simulink model "BasicAudio_Target"  (R2022b)
settings: Solver=FixedStepDiscrete  StartTime=0.0  StopTime=1  RelTol=1e-3  EnableMultiTasking=on
InitFcn:
  | % Initialize model
  | run([ ModelRootName() 'Init.m' ]);
  | 
  | % load library data
  | GainLibrary_data;
  | % Load saved values from partition process
  | TOP_Mask.LoadMapFromFile(bdroot)
model workspace (MAT data in the model file):
  PreampVolumeTable_Idx : Simulink.Signal (value not decoded)
  Range : Simulink.Signal (value not decoded)
  Table_Idx : Simulink.Signal (value not decoded)
undefined symbols (not defined in the file or in its folder): ModelCfg, RgainBusUtil
libraries: TOP x27, HandyTextFile x14, FeaturePath x7, SetDsm x6, RTC x5, AudioStats x3, CapturedConstLib x3, EdgePorts x2, MuteRamperBtc x1, RgainyBtc x1, simulink_need_slupdate x1, dspsrcs4 x1
(part 4 of 5)

== system BasicAudio_Target/BasicAudio/Treble/Tone/InnerLink/TuneVarOffset ==
  TOP : TOP/TOP  TriggerInit=[440 20 585 80]  TopName=Offset  DataTypeOut=single  BankNumber=BankNumber  PreOverlay=PreOverlay  PostOverlay=PostOverlay  CompatibilityString=[]  Role=Automatic
      settings: SourceProductName=Bose Talaria
  TrivialTranslation : Subsystem  mask(Talaria Trivial Translation){TriggerInit=[300 28 350 72]}
      mask prompts: TriggerInit "Hidden: MoveFcn redraw"
      mask help: A trivial translator connects to a TuneVar on the input side and to a TOP (Target Overlay Parameter) for output. The translator then simply copies the value from TuneVar to TOP with no changes.
      mask init:
      | TrivialTranslationMask.Init(gcbh);
      settings: MoveFcn=TrivialTranslationMask.CB_TriggerInit(gcbh);
      mask Callback TriggerInit: TrivialTranslationMask.CB_TriggerInit(gcbh);
      mask Display:
      | % retrieve icon definition
      | [path,w,h] = TrivialTranslationMask.Icon();
      | 
      | % retrieve the block's pixel size
      | pos = get(gcbh,'position');
      | bw = pos(3) - pos(1);
      | bh = pos(4) - pos(2);
      | 
      | % draw centered icon
      | xAdj = bw/2 - w/2;
      | yAdj = bh/2 - h/2;
      | for i=1:length(path)
      |    patch(path(i).x+xAdj, path(i).y+yAdj, path(i).rgb);
      | end
      | disp('COPY   ');
  Out1 : Outport  VectorParamsAs1DForOutWhenUnconnected=off
  wires:
  TOP/1 -> Out1/1  "variable"

== system BasicAudio_Target/BasicAudio/Treble/Tone/InnerLink/TuneVarRampTime ==
  TOP : TOP/TOP  TriggerInit=[440 20 585 80]  TopName=ramptime  DataTypeOut=single  BankNumber=BankNumber  PreOverlay=PreOverlay  PostOverlay=PostOverlay  CompatibilityString=[]  Role=Automatic
      settings: SourceProductName=Bose Talaria
  TrivialTranslation : Subsystem  mask(Talaria Trivial Translation){TriggerInit=[300 28 350 72]}
      mask prompts: TriggerInit "Hidden: MoveFcn redraw"
      mask help: A trivial translator connects to a TuneVar on the input side and to a TOP (Target Overlay Parameter) for output. The translator then simply copies the value from TuneVar to TOP with no changes.
      mask init:
      | TrivialTranslationMask.Init(gcbh);
      settings: MoveFcn=TrivialTranslationMask.CB_TriggerInit(gcbh);
      mask Callback TriggerInit: TrivialTranslationMask.CB_TriggerInit(gcbh);
      mask Display:
      | % retrieve icon definition
      | [path,w,h] = TrivialTranslationMask.Icon();
      | 
      | % retrieve the block's pixel size
      | pos = get(gcbh,'position');
      | bw = pos(3) - pos(1);
      | bh = pos(4) - pos(2);
      | 
      | % draw centered icon
      | xAdj = bw/2 - w/2;
      | yAdj = bh/2 - h/2;
      | for i=1:length(path)
      |    patch(path(i).x+xAdj, path(i).y+yAdj, path(i).rgb);
      | end
      | disp('COPY   ');
  Out1 : Outport  VectorParamsAs1DForOutWhenUnconnected=off
  wires:
  TOP/1 -> Out1/1  "variable"

== system BasicAudio_Target/BasicAudio/Treble/Tone/InnerLink/TuneVarScale ==
  TOP : TOP/TOP  TriggerInit=[440 20 585 80]  TopName=Scale  DataTypeOut=single  BankNumber=BankNumber  PreOverlay=PreOverlay  PostOverlay=PostOverlay  CompatibilityString=[]  Role=Automatic
      settings: SourceProductName=Bose Talaria
  TrivialTranslation : Subsystem  mask(Talaria Trivial Translation){TriggerInit=[300 28 350 72]}
      mask prompts: TriggerInit "Hidden: MoveFcn redraw"
      mask help: A trivial translator connects to a TuneVar on the input side and to a TOP (Target Overlay Parameter) for output. The translator then simply copies the value from TuneVar to TOP with no changes.
      mask init:
      | TrivialTranslationMask.Init(gcbh);
      settings: MoveFcn=TrivialTranslationMask.CB_TriggerInit(gcbh);
      mask Callback TriggerInit: TrivialTranslationMask.CB_TriggerInit(gcbh);
      mask Display:
      | % retrieve icon definition
      | [path,w,h] = TrivialTranslationMask.Icon();
      | 
      | % retrieve the block's pixel size
      | pos = get(gcbh,'position');
      | bw = pos(3) - pos(1);
      | bh = pos(4) - pos(2);
      | 
      | % draw centered icon
      | xAdj = bw/2 - w/2;
      | yAdj = bh/2 - h/2;
      | for i=1:length(path)
      |    patch(path(i).x+xAdj, path(i).y+yAdj, path(i).rgb);
      | end
      | disp('COPY   ');
  Out1 : Outport  VectorParamsAs1DForOutWhenUnconnected=off
  wires:
  TOP/1 -> Out1/1  "variable"

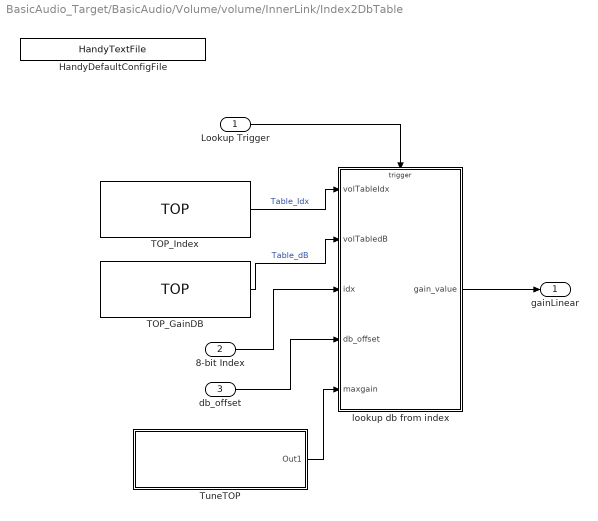
== system BasicAudio_Target/BasicAudio/Volume/volume/InnerLink/Index2DbTable ==
  Lookup Trigger : Inport
  8-bit Index : Inport  Port=2
  db_offset : Inport  Port=3
  HandyDefaultConfigFile : HandyTextFile/HandyTextFile  TemplateSource=Config  FileSuffix=Init  OpenDialogOnLoad=off  UseThisBlockName=off  AddGrandParentNamePrefix=off  TheDefaultText=|  ShowInLibBrowser=on
      | % $(FILENAME) Setup model parameters for each "Init" callback (e.g. update diagram)
      | sample_rate_in_hertz = 44100;
      | frame_size = 32;
      | sysin_channel_count = 2;
      settings: SourceProductName=Bose Talaria
  TOP_GainDB : TOP/TOP  TriggerInit=[635 177 785 233]  TopName=Table_dB  DataTypeOut=Inherit: Same as input  BankNumber=Config.BankNumber  PreOverlay=false  PostOverlay=false  CompatibilityString=[]  Role=Automatic
      settings: SourceProductName=Bose Talaria
  TOP_Index : TOP/TOP  TriggerInit=[635 97 785 153]  TopName=Table_Idx  DataTypeOut=Inherit: Same as input  BankNumber=Config.BankNumber  PreOverlay=false  PostOverlay=false  CompatibilityString=[]  Role=Automatic
      settings: SourceProductName=Bose Talaria
  TuneTOP : Subsystem  Description=Variable limits the maximum *dB offset* which will be applied to the gain as part of table lookup. It does *not* directly impact the maximum gain applied, only the maximum dB offset.  mask(Talaria Trivial Tune TOP){TriggerInit=[670 347 840 403], TopName=maxgain, DataTypeOut=single, BankNumber=0, PreOverlay=false, PostOverlay=false, UseSameName=on}
      mask prompts: TriggerInit "Hidden: MoveFcn redraw"; TopName "Name:"; DataTypeOut "Data type:"; BankNumber "Target memory bank number:"; PreOverlay "Requires pre-overlay action:"; PostOverlay "Requires post-overlay action:"; UseSameName "Use same name for tune variable and TOP"
      mask help: The TuneTOP block encapsultes a Target Overlay Parameter, a Tune Variable, and a Trivial Translation between them.
      mask init:
      | [ok,activeTopPath,activeTunePath] = TuneTOP_Mask.Init(gcbh);
      settings: MoveFcn=TuneTOP_Mask.CB_TriggerInit(gcbh);
      mask Callback TriggerInit: TuneTOP_Mask.CB_TriggerInit(gcbh);
      mask TypeOptions TopName: TOP/TopName
      mask TypeOptions DataTypeOut: TOP/DataTypeOut
      mask TypeOptions BankNumber: TOP/BankNumber
      mask TypeOptions PreOverlay: TOP/PreOverlay
      mask TypeOptions PostOverlay: TOP/PostOverlay
      mask Callback UseSameName: TuneTOP_Mask.CB_UseSameName(gcbh);
      mask DialogControl toolPanel Prompt: Tuning Tool Hints
      mask DialogControl DescriptionGroup Prompt: Description
      mask DialogControl DescriptionText Prompt: Variable limits the maximum *dB offset* which will be applied to the gain as part of table lookup. It does *not* directly impact the maximum gain applied, only the maximum dB offset.
      mask DialogControl EditDescription Prompt: Edit Description
      mask DialogControl EditDescription Callback: TuneTOP_Mask.CB_EditDescription(gcbh);
      mask DialogControl TunabilityText Prompt: Easy: Changes nearly every tuning.
      mask DialogControl AdvancedPanel Prompt: Advanced
      mask DialogControl ConvertToFullTranslation Prompt: Irreversible conversion to full translation
      mask DialogControl ConvertToFullTranslation Callback: TuneTOP_Mask.CB_ConvertToFullTranslation(gcbh);
      mask DialogControl ErrorContainer Prompt: Error Messages
      mask Display:
      | % retrieve icon definition
      | [path,w,h] = TuneTOP_Mask.Icon();
      | 
      | % retrieve the block's pixel size
      | pos = get(gcbh,'position');
      | bw = pos(3) - pos(1);
      | bh = pos(4) - pos(2);
      | 
      | % draw centered icon
      | xAdj = bw/2 - w/2 + 5;
      | yAdj = bh/2 - h/2 + 4;
      | for i=1:length(path)
      | 	patch(path(i).x+xAdj, path(i).y+yAdj, path(i).rgb);
      | end
      | 
      | % show the top name or an X
      | if (exist('ok','var') && ok)
      | 	text(bw*0.5, bh*0.2, activeTopPath, 'horizontalAlignment', 'center');
      | 	patch(0,0,[1 1 1]);
      | 	patch(bw,bh,[1 1 1]);
      | else
      | 	tx=bw*0.03;
      | 	ty=bh*0.03;
      | 	patch([0 tx bw bw-tx], [ty 0 bh-ty bh], [1 0 0]);
      | 	patch([0 bw-tx bw tx], [bh-ty 0 ty bh], [1 0 0]);
      | end
  lookup db from index : MATLAB Function  TreatAsAtomicUnit=on
  gainLinear : Outport  VectorParamsAs1DForOutWhenUnconnected=off
  wires:
  TuneTOP/1(Out1) -> lookup db from index/5(maxgain)
  db_offset/1 -> lookup db from index/4(db_offset)
  TOP_GainDB/1 -> lookup db from index/2(volTabledB)  "Table_dB"
  TOP_Index/1 -> lookup db from index/1(volTableIdx)  "Table_Idx"
  lookup db from index/1(gain_value) -> gainLinear/1
  Lookup Trigger/1 -> lookup db from index/Trigger
  8-bit Index/1 -> lookup db from index/3(idx)

== system BasicAudio_Target/BasicAudio/Volume/volume/InnerLink/Triggered Subsystem ==
  In1 : Inport
  Trigger : TriggerPort  TriggerType=function-call  VariantControl=Variant
  Out1 : Outport
  wires:
  In1/1 -> Out1/1

== system BasicAudio_Target/BasicAudio/Volume/volume/InnerLink/TuneVarRampTimeMs ==
  TOP : TOP/TOP  TriggerInit=[440 20 585 80]  TopName=RampTime  DataTypeOut=single  BankNumber=BankNumber  PreOverlay=PreOverlay  PostOverlay=PostOverlay  CompatibilityString=[]  Role=Automatic
      settings: SourceProductName=Bose Talaria
  TrivialTranslation : Subsystem  mask(Talaria Trivial Translation){TriggerInit=[300 28 350 72]}
      mask prompts: TriggerInit "Hidden: MoveFcn redraw"
      mask help: A trivial translator connects to a TuneVar on the input side and to a TOP (Target Overlay Parameter) for output. The translator then simply copies the value from TuneVar to TOP with no changes.
      mask init:
      | TrivialTranslationMask.Init(gcbh);
      settings: MoveFcn=TrivialTranslationMask.CB_TriggerInit(gcbh);
      mask Callback TriggerInit: TrivialTranslationMask.CB_TriggerInit(gcbh);
      mask Display:
      | % retrieve icon definition
      | [path,w,h] = TrivialTranslationMask.Icon();
      | 
      | % retrieve the block's pixel size
      | pos = get(gcbh,'position');
      | bw = pos(3) - pos(1);
      | bh = pos(4) - pos(2);
      | 
      | % draw centered icon
      | xAdj = bw/2 - w/2;
      | yAdj = bh/2 - h/2;
      | for i=1:length(path)
      |    patch(path(i).x+xAdj, path(i).y+yAdj, path(i).rgb);
      | end
      | disp('COPY   ');
  Out1 : Outport  VectorParamsAs1DForOutWhenUnconnected=off
  wires:
  TOP/1 -> Out1/1  "variable"

== system BasicAudio_Target/BasicAudio/Balance/balance/InnerLink/TuneVarBoostDisable/TrivialTranslation ==

== system BasicAudio_Target/BasicAudio/Balance/balance/InnerLink/TuneVarOffset/TrivialTranslation ==

== system BasicAudio_Target/BasicAudio/Balance/balance/InnerLink/TuneVarRampTime/TrivialTranslation ==

== system BasicAudio_Target/BasicAudio/Balance/balance/InnerLink/TuneVarSilentBass/TrivialTranslation ==

== system BasicAudio_Target/BasicAudio/Balance/balance/InnerLink/TuneVarSilentExtreme/TrivialTranslation ==

== system BasicAudio_Target/BasicAudio/Bass/Tone/InnerLink/TuneVarOffset/TrivialTranslation ==

== system BasicAudio_Target/BasicAudio/Bass/Tone/InnerLink/TuneVarRampTime/TrivialTranslation ==

== system BasicAudio_Target/BasicAudio/Bass/Tone/InnerLink/TuneVarScale/TrivialTranslation ==

== system BasicAudio_Target/BasicAudio/Mute/mute/InnerLink/MuteControl/Triggered Subsystem ==
  In1 : Inport
  Trigger : TriggerPort  TriggerType=function-call  VariantControl=Variant
  Out1 : Outport
  wires:
  In1/1 -> Out1/1

== system BasicAudio_Target/BasicAudio/Mute/mute/InnerLink/MuteControl/TuneVarRampTime ==
  TOP : TOP/TOP  TriggerInit=[440 20 585 80]  TopName=RampTime  DataTypeOut=single  BankNumber=BankNumber  PreOverlay=PreOverlay  PostOverlay=PostOverlay  CompatibilityString=[]  Role=Automatic
      settings: SourceProductName=Bose Talaria
  TrivialTranslation : Subsystem  mask(Talaria Trivial Translation){TriggerInit=[300 28 350 72]}
      mask prompts: TriggerInit "Hidden: MoveFcn redraw"
      mask help: A trivial translator connects to a TuneVar on the input side and to a TOP (Target Overlay Parameter) for output. The translator then simply copies the value from TuneVar to TOP with no changes.
      mask init:
      | TrivialTranslationMask.Init(gcbh);
      settings: MoveFcn=TrivialTranslationMask.CB_TriggerInit(gcbh);
      mask Callback TriggerInit: TrivialTranslationMask.CB_TriggerInit(gcbh);
      mask Display:
      | % retrieve icon definition
      | [path,w,h] = TrivialTranslationMask.Icon();
      | 
      | % retrieve the block's pixel size
      | pos = get(gcbh,'position');
      | bw = pos(3) - pos(1);
      | bh = pos(4) - pos(2);
      | 
      | % draw centered icon
      | xAdj = bw/2 - w/2;
      | yAdj = bh/2 - h/2;
      | for i=1:length(path)
      |    patch(path(i).x+xAdj, path(i).y+yAdj, path(i).rgb);
      | end
      | disp('COPY   ');
  Out1 : Outport  VectorParamsAs1DForOutWhenUnconnected=off
  wires:
  TOP/1 -> Out1/1  "variable"

== system BasicAudio_Target/BasicAudio/Treble/Tone/InnerLink/TuneVarOffset/TrivialTranslation ==

== system BasicAudio_Target/BasicAudio/Treble/Tone/InnerLink/TuneVarRampTime/TrivialTranslation ==

== system BasicAudio_Target/BasicAudio/Treble/Tone/InnerLink/TuneVarScale/TrivialTranslation ==

== system BasicAudio_Target/BasicAudio/Volume/volume/InnerLink/Index2DbTable/TuneTOP ==
  TOP : TOP/TOP  TriggerInit=[440 20 585 80]  TopName=maxgain  DataTypeOut=single  BankNumber=BankNumber  PreOverlay=PreOverlay  PostOverlay=PostOverlay  CompatibilityString=[]  Role=Automatic
      settings: SourceProductName=Bose Talaria
  TrivialTranslation : Subsystem  mask(Talaria Trivial Translation){TriggerInit=[300 28 350 72]}
      mask prompts: TriggerInit "Hidden: MoveFcn redraw"
      mask help: A trivial translator connects to a TuneVar on the input side and to a TOP (Target Overlay Parameter) for output. The translator then simply copies the value from TuneVar to TOP with no changes.
      mask init:
      | TrivialTranslationMask.Init(gcbh);
      settings: MoveFcn=TrivialTranslationMask.CB_TriggerInit(gcbh);
      mask Callback TriggerInit: TrivialTranslationMask.CB_TriggerInit(gcbh);
      mask Display:
      | % retrieve icon definition
      | [path,w,h] = TrivialTranslationMask.Icon();
      | 
      | % retrieve the block's pixel size
      | pos = get(gcbh,'position');
      | bw = pos(3) - pos(1);
      | bh = pos(4) - pos(2);
      | 
      | % draw centered icon
      | xAdj = bw/2 - w/2;
      | yAdj = bh/2 - h/2;
      | for i=1:length(path)
      |    patch(path(i).x+xAdj, path(i).y+yAdj, path(i).rgb);
      | end
      | disp('COPY   ');
  Out1 : Outport  VectorParamsAs1DForOutWhenUnconnected=off
  wires:
  TOP/1 -> Out1/1  "variable"

== system BasicAudio_Target/BasicAudio/Volume/volume/InnerLink/TuneVarRampTimeMs/TrivialTranslation ==

== system BasicAudio_Target/BasicAudio/Mute/mute/InnerLink/MuteControl/TuneVarRampTime/TrivialTranslation ==

== system BasicAudio_Target/BasicAudio/Volume/volume/InnerLink/Index2DbTable/TuneTOP/TrivialTranslation ==

== matlab function BasicAudio_Target/BasicAudio/Balance/balance/InnerLink/balanceProcess ==
  data: audioIn input; audioOut output; channelToRamperMap input; Rampers data_store_memory; Freeze data_store_memory; MaskNumRampers parameter
function audioOut  = balanceProcess(audioIn, channelToRamperMap, ... % inputs
    MaskNumRampers)  % parameters

% Applies the Left and Right gains to the respective channels via multiple
%   rampers
% Inputs:
%  audioIn: Input audio
%  channelToRamperMap: Input channels mapped to their corresponding ramper.
%  MaskNumRampers: Number of rampers (set in the Mask file) = 4

% Data Store objects (registered in "Edit Data" dialog)
global Rampers;
global Freeze;

% Figure out the frame size, channel count and number of rampers
[frameSize, ~] = size(audioIn);

% set the size and datatype of the output buffer
audioOut = coder.nullcopy(audioIn);

%   Every channel needs a ramper, but every ramper does not need to be on a
%   channel necessarily.
for ramper = 1:MaskNumRampers
    % Get the gains
    gain = Rampers(ramper).currentGain;
    rampCoeffMultipliers = ones(1, frameSize, 'single');
    if (Freeze(1) == false)
        if (Rampers(ramper).frameCount == 0)
            % The ramp is finished. Stop ramping and SNAP to the target
            gain = Rampers(ramper).targetGain;
        else
            % The ramp is *NOT* frozen or done: gain is moving
            k = Rampers(ramper).rampCoeff;
            rampCoeffMultipliers = (k * rampCoeffMultipliers) .^ (1:frameSize);
            Rampers(ramper).frameCount = Rampers(ramper).frameCount - 1;
        end
    end
    
    % Apply the gains to the corresponding channels via the Mask parameter
    % and tuneTop paramter "channelToRamperMap".  
    currentChannelGroup = find(channelToRamperMap == ramper);
    for ch = 1:numel(currentChannelGroup)
        audioOut(:,currentChannelGroup(ch)) = (gain * rampCoeffMultipliers)' .* audioIn(:,currentChannelGroup(ch));
    end
    Rampers(ramper).currentGain = gain * rampCoeffMultipliers(end);
end

% If ramper value of -1 is encountered, this indicates an unused channel.
% Assign values of zero to all samples of these channels.
unusedChannelGroup = find(channelToRamperMap == -1);
for unusedCh = 1:numel(unusedChannelGroup)
    audioOut(:,unusedChannelGroup(unusedCh)) = 0;
end

== matlab function BasicAudio_Target/BasicAudio/Balance/balance/InnerLink/calculate_balance_gain ==
  data: balanceIndex input; balanceTableDb input; balanceTableIdx input; indexOffset input; boostDisable input; EnableSilentExtreme input; SleepingBeautyMutesBass input; targetGains output; MaskNumRampers parameter
  events: trigger input FUNCTION_CALL_EVENT
function targetGains  = Calculate_Balance_Gain(balanceIndex, ...
    balanceTableDb, balanceTableIdx, ...
    indexOffset, boostDisable, EnableSilentExtreme, SleepingBeautyMutesBass, MaskNumRampers)

% Computes the balance gains for the 'left' and 'right' channel groups. 
% Based on the position of the balance index in 'balanceTableIdx', the 
% corresponding 'cut' gain is computed from the 'balanceTableDb'. If the 
% index lies between two entries in the table, the gain is computed by 
% linear interpolation between the corresponding gain table entries. 
% The 'boost' gain is computed based from the 'cut' gain depending on the
% value of the tune variable, 'boostDisable'. If set to '1', boost is 0 dB 
% and if '0', in order to preserve energy, the boost is computed based on
% the following equation: Boost^2 + Cut^2 = 2. 
% If 'silent extreme' is enabled and the index at either extreme is
% requested, channels belonging to the group which receives a gain 'cut'
% are muted.

j = uint8(1);
cut_linear = single(0.0);

targetGains = coder.nullcopy(ones(1,MaskNumRampers,'single'));
balanceIndex = single(balanceIndex);
% random comment


% Find the left and the right gains
% Based on the balance table, the dB value of the index is calculated
while (j <= numel(balanceTableIdx))
    if (balanceIndex <= balanceTableIdx(j))
        if (j <= 1)  % first indexed value is linearly interpolated to zero
            if (balanceTableIdx(j))
                percent = balanceIndex / balanceTableIdx(j);
            else
                percent = single(1);
            end
            cut_linear = percent * 10 ^ (balanceTableDb(j) / 20);
        else         % other values are interpolated in db space
            lastIdx = single(balanceTableIdx(j-1));
            percent = (balanceIndex - lastIdx) / (balanceTableIdx(j) - lastIdx);
            cut_linear = 10 ^ (((percent * (balanceTableDb(j) - balanceTableDb(j-1))) + balanceTableDb(j-1)) / 20);
        end
        break;
    else
        j = j + 1;
    end
end

% Boost of > 0 dB is dependant on tuning. If the tune variable is SET (1),
% boost of 0 dB is applied (i.e. linear value of 1). If the tune variable
% is RESET (0), a boost of 3 dB is applied
if boostDisable == 0
    boost_linear = sqrt(2.0 - cut_linear^2);
else
    boost_linear = single(1);
end

% % if silent extreme is enabled and we're extreme, make the cut complete
% % (Sleeping Beauty)
if (EnableSilentExtreme && abs(balanceIndex - indexOffset) >= (indexOffset-1))
    cut_linear = single(0);
end

% Assign left and right Gain Values
if (balanceIndex - indexOffset) > 0 % Left speakers attenuated
    left = single(cut_linear);
    right = single(boost_linear);
else
    left = single(boost_linear);
    right = single(cut_linear);
end

% Assign remaining gain values 
center = (left + right) * 0.5;
mono = center;

% Number to Content Key
targetGains(1) = left;
targetGains(2) = right;
targetGains(3) = center;
targetGains(4) = mono;

% (Sleeping Beauty)
% if silent extreme is enabled and we're extreme, cut center freqs
if (EnableSilentExtreme && abs(balanceIndex - indexOffset) >= (indexOffset-1))
    targetGains(3) = 0;
    if (SleepingBeautyMutesBass)
        targetGains(4) = 0;
    end
end

== matlab function BasicAudio_Target/BasicAudio/Balance/balance/InnerLink/calculate_ramp_parameters ==
  data: rampTimeTune input; rampRateRTC input; rampTimeRTC input; ramptime output; rampRate output; rampRateBounds parameter; rampTimeBounds parameter
  events: trigger input FUNCTION_CALL_EVENT
function [ramptime, rampRate]  = calculate_ramp_parameters(...
    rampTimeTune, rampRateRTC,rampTimeRTC, ... % inputs
    rampRateBounds, rampTimeBounds) % parameters

% Ramp time and rate are provided to the block through RTC messages. However 
% in case neither of them are provided, the block will use the default ramp 
% time given in the tune variables.

    ramptime = single(rampTimeTune);
    rampRate = single(0);

    if (rampRateRTC)
        rampRate = single(rampRateRTC);
        rampRate = max(rampRateBounds(1), rampRate);
        rampRate = min(rampRateBounds(2), rampRate);
    end
    if (rampTimeRTC)
        ramptime = single(rampTimeRTC);
    end
    ramptime = max(rampTimeBounds(1), ramptime);
    ramptime = min(rampTimeBounds(2), ramptime);
end

== matlab function BasicAudio_Target/BasicAudio/Balance/balance/InnerLink/check sequence ==
  data: done output; Rampers data_store_memory; MaskNumRampers parameter
  events: trigger input FUNCTION_CALL_EVENT
function done = GetCompletedSequence(MaskNumRampers)
% Function which checks if the notification sequence
% has completed successfully 

global Rampers;

% Assume the work is complete until proven otherwise
done = true;

for i=1:MaskNumRampers
   if (Rampers(i).targetGain ~= Rampers(i).currentGain)
       done = false; % just proved otherwise
       break;
   end
end

== matlab function BasicAudio_Target/BasicAudio/Balance/balance/InnerLink/control ==
  data targetGainLinear settings: description=This vector signal must provide a linear target gain for every ramper.
  data rampdbPerSec settings: description="If provided (i.e. non zero), this argument causes the \"ramp times (ms)\" input to be ignored. The block will calculate ramp times itself to ensure all gain changes happen at the db_per_sec slope provided."
  data rampTimesMs settings: description=|
      | The rampTimes_ms signal can accept one or more ramp times. If only one time is given, it is applied to all rampers. When more than one time is given, the times are delt out to the rampers in order. If not enough times are specified to cover all the rampers, the last given time is filled in to any remaining rampers.
      | NOTE: this input signal is entirely ignored if the db_per_sec input signal is non-zero. Attach the db_per_sec input to a ground block if you want to provide ramp times via this input.
  data sampleRateInHertz settings: description="This input is required for control calculations to work. The \"Audio Stats\" block is a handy tool to lift this property right off an inbound audio signal and feed it to this block automatically without using workspace parameters or other constants."
  data frameSize settings: description="This input is required for control calculations to work. The \"Audio Stats\" block is a handy tool to lift this property right off an inbound audio signal and feed it to this block automatically without using workspace parameters or other constants."
  data: targetGainLinear input size=[1 MaskNumRampers]; rampdbPerSec input; rampTimesMs input; sampleRateInHertz input; frameSize input; Rampers data_store_memory; MaskNumRampers parameter
  events: trigger input FUNCTION_CALL_EVENT
function control(...
     targetGainLinear, rampdbPerSec, rampTimesMs, sampleRateInHertz, ...
     frameSize, ... % inputs
     MaskNumRampers) % parameters
%#codegen
% CONTROL LOGIC:
% Shift of 'balance' between the 'Right' and 'Left' channel groups is
% achieved by multiplying the corresponding 'cut' or 'boost' gain. As the
% index increases from 0, the balance shifts from left to right. Channels
% corresponding to the 'center' group are not modified. 
% rampdbPerSec takes precidence:
% If dbPerSec has a non-zero value then any ramp_times_ms values are
% ignored and the dbPerSec is used to determine ramper timing.
% Inputs:
%   targetGainLinear: Indicates the gain (in linear scale) which needs to
%       be applied to the audio. Gain values can be mapped to the ramper
%       configuration.
%   rampTimeMs: Indicates the time in milliseconds in which the gain of the
%       rampers must change from their current to target values.
%   rampdbPerSecond: Indicates the rate in dB/second at which the gain of the
%       rampers must change from their current to target values. If this
%       value is non-zero, it is used to compute the ramp time and
%       'rampTimeMs' is discarded (if specified).
%   rgain_SILENT_GAIN: Parameter defined in the initFcn callback.

% Control Data:
%   Freeze(1) freezes the processing during this control operation
%   Rampers(1) is the ramper for the 'Left' group. Boost vs. cut 
%        is determined by the value of the balance index.
%   Rampers(2) is the ramper for the 'Right' group. Boost vs. cut is determined by
%        the value of the balance index.
%   Rampers(3) is the ramper for the 'Center' group. Boost vs. cut is determined by
%        the value of the balance index.
%   Rampers(4) is the ramper for the 'Mono' group (supporting "Sleeping
%       Beauty Mutes Bass"). Boost vs. cut is determined by the value of 
%       the balance index.

global Rampers;

% Step 1: FREEZE the gain ramper so that we can perform calculations based
% on the current gain value. (This step is done outside on canvas now)

% This block replaces much of rgainy, but uses its own silent gain value.
% The reason why is not documented, but it does impact all the test cases.
% Use this special value instead of RgainBusUtil.GetSilentGainLinear
rgain_SILENT_GAIN = single(10^(-126/20));

% Step 2: Nudge the gain values a bit if they are sitting at zero.
% When this control set goes live, ensure that the current gain will move.
% If current gain is zero, replace with a value very close to zero. What we
% really want is a value which is on the edge of perception - not too small
% or large. If the value is too small, we'll waste some of our ramp time
% in perceived silence. If the value is too large, the audio will lurch
% into perceptability at the start of the ramp.
% UPDATE: This will now loop over 4 rampers

currentGainLinear = zeros(1,MaskNumRampers,'single');
for i = 1:MaskNumRampers
    currentGainLinear(i) = max(Rampers(i).currentGain, rgain_SILENT_GAIN);
    targetGainLinear(i) = max(targetGainLinear(i), rgain_SILENT_GAIN);
end

% Step 3a: If a slope in dB/second is provided, ignore the ramp time
% and instead calculate a new ramp time that matches the slope.
rampMs = zeros(1,MaskNumRampers,'single');
if (rampdbPerSec)
    currentGainDb = 20*log10(currentGainLinear);
    targetGainDb = 20*log10(targetGainLinear);
    diff = abs(currentGainDb - targetGainDb);
    rampMs = diff / single(rampdbPerSec) * 1000;
else
    rampMs(:) = single(rampTimesMs);
end
    
% Step 3b: QUANTIZE the desired ramp time to our FrameSize. Also retrieve 
% the whole number of frames required to best match requested ramp time.
% Ensure that at least one frame is used. The frame size will therefore
% determine the steepest ramp (i.e. within one frame you can go anywhere).
quantumMs = 1000 * frameSize / sampleRateInHertz;
numFrames = rampMs / quantumMs;
numFrames = max (1, ceil(numFrames));
quantizedRampTimeMs = numFrames * quantumMs;

% UPDATE: Loop over 4 rampers now (L, R, C, and Mono)
for ramper=1:MaskNumRampers
    % In order to have the desired ramp time, the slope must vary dependent
    % on the gain differencebetween target and current value.
    % Ramper's coefficient is therefore calculated as follows:
    %
    %   TargetGain = CurrentGain *( RampCoef ^ (Fs*RampTime_ms/1000) )
    %
    % therefore...
    %
    %                     log(TargetGain/CurrentGain)
    %   log(RampCoef) = ------------------------------
    %                        Fs*(RampTime_ms/1000)
    %
    factor = log( targetGainLinear(ramper) / currentGainLinear(ramper) );
    RampCoef = double(exp(factor / (sampleRateInHertz * quantizedRampTimeMs(ramper) / 1000)));
    
    % Output control signals
    Rampers(ramper).frameCount  = int32(numFrames(ramper));    
    Rampers(ramper).targetGain  = targetGainLinear(ramper);
    Rampers(ramper).rampCoeff = single(RampCoef);
    Rampers(ramper).currentGain = currentGainLinear(ramper);
end
% unfreeze the gain (This step is done outside on canvas now)

== matlab function BasicAudio_Target/BasicAudio/Mute/mute/InnerLink/MuteControl/calculate_ramp_rate ==
  data: rampRateRTC input; rampRate output; rampTimeRTC input; ramptime output; rampTimeTune input; rampRateBounds parameter; rampTimeBounds parameter
  events: trigger input FUNCTION_CALL_EVENT
function [rampRate,ramptime] = Calculate_ramp_parameters(rampRateRTC, rampTimeRTC, rampTimeTune,... % Inputs
    rampRateBounds, rampTimeBounds) % parameters

% Ramp time and rate are provided to the block through RTC messages. However 
% in case neither of them are provided, the block will use the default ramp 
% time given in the tune variable.

    ramptime = single(rampTimeTune);
    rampRate = single(0);
    
    if (rampRateRTC)
        rampRate = single(rampRateRTC);
        rampRate = max(rampRateBounds(1), rampRate);
        rampRate = min(rampRateBounds(2), rampRate);
    end
    if (rampTimeRTC)
        ramptime = single(rampTimeRTC);
    end
    ramptime = max(rampTimeBounds(1), ramptime);
    ramptime = min(rampTimeBounds(2), ramptime);
end

== matlab function BasicAudio_Target/BasicAudio/Treble/Tone/InnerLink/check done ==
  data: done output; Rampers data_store_memory
  events: trigger input FUNCTION_CALL_EVENT
function done  = fcn
%#codegen

global Rampers;

% Checking whether the frameCounts are exactly equal to 0 was leading to
% unpredictable behavior. Therefore, we now check whether or not the 
% frameCounts are less-than/equal-to 0.
% See SAMPLERATE-1196 & SAMPLERATE-1205 for more details. 
done = (Rampers(1).frameCount <= 0) && (Rampers(2).frameCount <= 0);

== matlab function BasicAudio_Target/BasicAudio/Treble/Tone/InnerLink/index to linear ==
  data: linearGain output; scale input; offset input; index input
  events: trigger input FUNCTION_CALL_EVENT
function linearGain = compute_gain(scale,offset,index)
%#codegen

% The midrange curve is configured as a piecewise linear plot, with
% configurable values of the maximum boost ('maxB') and maximum cut ('maxC')
% in dB. 
%    dB ^
%       |
% maxB  ----------/
%       |        /
%       |       /
%  0    ------|---|----> index
%       |   /128  255
%       |  /
% maxC  --/
%       |
% Hence, for any given index, the gain is calculated as a value in 
% between 0 and 1 for boost and 0 and -1 for cut. This will later be
% multiplied with the maxB or maxC to get the actual gain value. 
% (y - y1) / (x - x1) = (y1 - y2) / (x1 - x2)
% (y - 0) / (x - 128) = (0 - 1) / (128 - 255)
%                   y = (x - 128)/127
% 'offset' represents the center point between boost and cut (i.e. 128) and
% 'scale' represents how many intervals are available for boost/cut (i.e. 127)

% Apply the tuning calibration
floatIndex = single(index);
linearGain = single((floatIndex - offset) / scale);

% Ensure the result is between -1 and 1
linearGain = min(linearGain, 1);
linearGain = max(linearGain, -1);

== matlab function BasicAudio_Target/BasicAudio/Treble/Tone/InnerLink/ramp parameters ==
  data: data input; ramptime output; rampTimeRTC input; rampRateRTC input; rampRate output; rampRateBounds parameter; rampTimeBounds parameter
  events: trigger input FUNCTION_CALL_EVENT
function [ramptime, rampRate]  = ramp_parameters( data, rampTimeRTC, rampRateRTC,... % inputs
    rampRateBounds, rampTimeBounds) % parameters

%#codegen
    % Ramp time mentioned in the RTC message gets priority over the tune
    % variable. Boundary conditions are also included based on BDSP values.
    % If neither ramp time nor rate are given in the RTC message (i.e. both
    % = 0), then the ramp time in the Tune variable is taken as the default
    % value for that message.
    
    ramptime = single(data);
    rampRate = single(0); 
    
    if (rampRateRTC)
        rampRate = single(rampRateRTC);
        rampRate = max(rampRateBounds(1), rampRate);
        rampRate = min(rampRateBounds(2), rampRate);
    end
    if (rampTimeRTC)
        ramptime = single(rampTimeRTC);
    end
    ramptime = max(rampTimeBounds(1), ramptime);
    ramptime = min(rampTimeBounds(2), ramptime);
end

== matlab function BasicAudio_Target/BasicAudio/Treble/Tone/InnerLink/tone ==
  data: audioOut output; boost_coeffs input; cut_coeffs input; audioIn input; Rampers data_store_memory; gain output; Freeze data_store_memory; Phase data_store_memory
function [audioOut,gain] ...
    = toneProcess(boost_coeffs, cut_coeffs, audioIn)...    % inputs % parameters
  
%#codegen

% Data Store objects (registered in "Edit Data" dialog
global Rampers;
global Freeze;
global Phase;

% Keep memory for the filter persistent from frame to frame
persistent toneFilterStates;

% figure out the frame size and channel count
[frame_size, channel_count] = size(audioIn);

if (isempty(toneFilterStates))
    toneFilterStates = zeros(1,channel_count,'single');
end


% set the size and datatype of the output buffer
audioOut = coder.nullcopy(audioIn);

ramper = Phase;
ramperCount = numel(Rampers);

if (Freeze == false)
    if (Rampers(ramper).frameCount == 0)
        % The current ramper is finished. Is there another one?
        if (ramper < ramperCount && Rampers(ramper+1).frameCount > 0)
            % Yes - move on to the next phase
            ramper = ramper + 1;
            Phase = ramper;
            k = Rampers(ramper).rampCoeff;
            gain = Rampers(ramper).currentGain;
            Rampers(ramper).frameCount = Rampers(ramper).frameCount - 1;
        else
            %  Stop ramping and SNAP to the target
            k = single(1);
            gain = Rampers(ramper).targetGain;
            % Update completion flag
         end
    else
        % The ramp is *NOT* frozen or done: gain is moving
        k = Rampers(ramper).rampCoeff;
        gain = Rampers(ramper).currentGain;
        Rampers(ramper).frameCount = Rampers(ramper).frameCount - 1;
    end
else
    % Frozen. Stay at current gain
    k = single(1);
    gain = Rampers(ramper).currentGain;
end

% Apply the tone filter
if (gain < 1)
    % Cut
    bCoeffs = cut_coeffs(1:2);
    aCoeffs = cut_coeffs(3);
else
    % Boost
    bCoeffs = boost_coeffs(1:2);
    aCoeffs = boost_coeffs(3);
end

% [filtered,toneFilterStates] = filter(bCoeffs, aCoeffs, audioIn, toneFilterStates);

% Loop through samples, adjusting gain and applying to channels
for n=1:frame_size
    % Update the gain and then subtract one before applying it to the
    % filtered signal. Disregarding phase shifting 
    gain = gain * k;
    filterGain = gain - 1;
    % Loop through channels adding in gain-adjusted filtered samples
    for chanIdx = 1:channel_count
        
        filterOut = (bCoeffs(1) * audioIn(n,chanIdx)) + toneFilterStates(chanIdx);
        toneFilterStates(chanIdx) = (bCoeffs(2) * audioIn(n,chanIdx)) + (aCoeffs(1) * filterOut);
        
        audioOut(n,chanIdx) = audioIn(n,chanIdx) + (filterOut * filterGain);
    end
end

Rampers(ramper).currentGain = gain;

== matlab function BasicAudio_Target/BasicAudio/Treble/Tone/InnerLink/tone control ==
  data normalized_gain_impact settings: description=This vector signal must provide a linear target gain for every ramper.
  data db_per_sec settings: description="If provided (i.e. non zero), this argument causes the \"ramp times (ms)\" input to be ignored. The block will calculate ramp times itself to ensure all gain changes happen at the db_per_sec slope provided."
  data ramp_time_ms settings: description=|
      | The rampTimes_ms signal can accept one or more ramp times. If only one time is given, it is applied to all rampers. When more than one time is given, the times are delt out to the rampers in order. If not enough times are specified to cover all the rampers, the last given time is filled in to any remaining rampers.
      | NOTE: this input signal is entirely ignored if the db_per_sec input signal is non-zero. Attach the db_per_sec input to a ground block if you want to provide ramp times via this input.
  data sample_rate_in_hertz settings: description="This input is required for control calculations to work. The \"Audio Stats\" block is a handy tool to lift this property right off an inbound audio signal and feed it to this block automatically without using workspace parameters or other constants."
  data frame_size settings: description="This input is required for control calculations to work. The \"Audio Stats\" block is a handy tool to lift this property right off an inbound audio signal and feed it to this block automatically without using workspace parameters or other constants."
  data: boost_max_db input; cut_max_db input; normalized_gain_impact input size=1; db_per_sec input; ramp_time_ms input; sample_rate_in_hertz input; frame_size input; Rampers data_store_memory; rgain_SILENT_GAIN parameter; Phase data_store_memory
  events: trigger input FUNCTION_CALL_EVENT
function control(...
    boost_max_db, cut_max_db, ... %inputs
    normalized_gain_impact, db_per_sec, ramp_time_ms, sample_rate_in_hertz, frame_size, ... % inputs % parameters
    rgain_SILENT_GAIN) %parameters

% See Control summary at the end:
global Phase;
global Rampers;

% Step 1: FREEZE the gain ramper so that we can perform calculations based
% on the current gain value. (This step now performed on canvas)

% Step 2a: IMPACT-TARGET Translate the normalized gain into a dB impact
% based on the maximum boost or cut values.
% ("-1" = maximum cut, "1" = maximum boost.)
targetIsBoost = (normalized_gain_impact >= 0);
if (targetIsBoost)
    targetImpact_db = normalized_gain_impact * boost_max_db;
    targetEffectiveGain = undb20(targetImpact_db); % 1 or greater
else
    targetImpact_db = normalized_gain_impact * cut_max_db;
    targetEffectiveGain = undb20(targetImpact_db); % less than 1
end

actualTargetGainLinear = targetEffectiveGain; 

% Step 2b: IMPACT-CURRENT Fetch the current gain from the previously
% active ramper.
currentPhase = Phase;
currentGain = Rampers(currentPhase).currentGain;
currentIsBoost = (currentGain >= 1);
currentImpact_db = db20(currentGain);

% Setup processing to continue on seamlessly while we work here
Rampers(1).currentGain = currentGain;
Phase = uint32(1); % reset phase to 1
% Now that we have both current and target impacts, find the difference
db_diff = abs(currentImpact_db - targetImpact_db);

% Step 3a: TIME- If a slope in dB/second is provided, ignore the ramp time
if (db_per_sec)
    ramp_ms = db_diff / single(db_per_sec) * 1000;
else
    ramp_ms = single(ramp_time_ms);
end
    
% Step 3b: TIME- QUANTIZE the desired ramp time to our FrameSize. 
quantum_ms = 1000 * frame_size / sample_rate_in_hertz;
numFrames = ramp_ms / quantum_ms;
numFrames = max (1, ceil(numFrames));

% Step 4a: PHASES- Determine whether ramping from current gain to target
% gain requires a unity crossing in linear gain.
isTwoPhase = (currentIsBoost ~= targetIsBoost) && ...
             (currentGain ~= 1) && ... % cannot cross if you're already there
             (targetImpact_db ~= 1);  % no crossing needed when impact already nothing
% Setup a structure to hold information about what the rampers should do
twoSingles = {single(0) single(0)};
phaseConfig = struct('frames',twoSingles,'target_linear',twoSingles,'current_linear',twoSingles);
phaseConfig = tone_control_split(numFrames,currentImpact_db,db_diff,...
    currentGain,currentIsBoost,rgain_SILENT_GAIN,targetIsBoost,...
    targetEffectiveGain,isTwoPhase,phaseConfig);

% Step 4b: PHASES- Setup rampers for both phases
for currentPhase=1:2
    if (phaseConfig(currentPhase).frames)
        ramp_ms = quantum_ms * phaseConfig(currentPhase).frames;
        factor = log(phaseConfig(currentPhase).target_linear / phaseConfig(currentPhase).current_linear);
        RampCoef = exp(factor / (sample_rate_in_hertz * ramp_ms / 1000));
    else
        RampCoef = single(1);
    end
    Rampers(currentPhase).rampCoeff   = single(RampCoef);
    Rampers(currentPhase).targetGain  = actualTargetGainLinear; % phase 1 value ignored.
    Rampers(currentPhase).currentGain = single(phaseConfig(currentPhase).current_linear);
    Rampers(currentPhase).frameCount  = int32(phaseConfig(currentPhase).frames);
end

% unfreeze the gain. (This step now performed on canvas)


end

% Nudge the gain values a bit if they are sitting right at one (aka unity).
% When a control set goes live, ensure that the current gain will move.
% If current gain is one, replace with a value very close to one. What we
% really want is a value which is on the edge of perception - not too small
% or large. If the value is too small, we'll waste some of our ramp time
% in perceived silence. If the value is too large, the audio will lurch
% into perceptability at the start of the ramp. Remember that normally we
% worry about gains of 0 -- this checks instead against 1 because filter
% gain is effective gain minuus 1.
function adjustedLinearGain = NudgeUnity(linearGain,isPositive,silentGain)
    if (isPositive)
        adjustedLinearGain = max(linearGain, 1 + silentGain);
    else
        adjustedLinearGain = min(linearGain, 1 - silentGain);
    end
end

function phaseConfig = tone_control_split(numFrames,currentImpact_db,db_diff,...
    currentGain,currentIsBoost,rgain_SILENT_GAIN,targetIsBoost,...
    targetEffectiveGain,isTwoPhase,phaseConfig)
if (isTwoPhase)
    % Both boost and cut phases will be required to get where we are going.
    % Make sure we have at least two frames to work with:
    numFrames = max (2, round(numFrames));
    
    % Divide up our ramp time into pieces for each phase to use
    phase1Frames = ceil(numFrames * abs(currentImpact_db) / db_diff);
    phase2Frames = numFrames - phase1Frames;
    
    % Make sure phase 2 has at least 1 frame to work with
    phase2Frames = max(1, phase2Frames);
    
    % Setup Phase 1 ramper that takes us to zero impact (i.e. unity gain)
    phaseConfig(1).current_linear   = currentGain;  % we know this is not 1
    phaseConfig(1).target_linear    = NudgeUnity(1,currentIsBoost,rgain_SILENT_GAIN);
    phaseConfig(1).frames           = phase1Frames;
    
    % Setup Phase 2 ramper that delivers us to target impact
    phaseConfig(2).current_linear   = NudgeUnity(1,targetIsBoost,rgain_SILENT_GAIN); % start quiet
    phaseConfig(2).target_linear    = targetEffectiveGain;   % we know this is not 0
    phaseConfig(2).frames           = phase2Frames;
else
    % Only one phase is needed to accomplish our goal. We are are the
    % target side of unity... but we must determine which side that is
    if (currentGain == 1)
        % One is in-between sides: use the target to determine the side
        isBoost = targetIsBoost;
    else
        % Current gain is already on one side of unity so use that
        isBoost = currentIsBoost;
    end
    phaseConfig(1).current_linear   = NudgeUnity(currentGain,isBoost,rgain_SILENT_GAIN);
    phaseConfig(1).target_linear    = NudgeUnity(targetEffectiveGain,isBoost,rgain_SILENT_GAIN);
    phaseConfig(1).frames           = numFrames;
    
    % Setup Phase 2 ramper to sit at the target gain
    phaseConfig(2).current_linear   = NudgeUnity(targetEffectiveGain,isBoost,rgain_SILENT_GAIN);
    phaseConfig(2).target_linear    = NudgeUnity(targetEffectiveGain,isBoost,rgain_SILENT_GAIN);
    phaseConfig(2).frames           = single(0);
end
end

% This routine sets up the control data that directs the operation of
% the signal processing logic. The high level design of the tone block
% involves filtering out frequency range of the signal and then mixing it
% back in. This results in a boost or a cut to the filtered frequencies. As
% such, the gain of the filtered signal equals the overall tone block's
% effective gain minus 1 for the unfiltered signal.
%
% FilterGain = EffectiveGain - 1
%                             _
%                            / \   EffectiveGain
%   >-------+-------------->| + |------------------>
%           |                \ /
%           v                 |
%      +----+---+             ^
%      |        |            / \
%      | Filter |           /   \ FilterGain
%      |        |          /gain \
%      +----+---+          +-----+
%           |                 ^
%           |                 |
%           +-----------------+
%
% Another issue of note is that crossing over from boost to cut or vice
% versa involves numerically crossing 0 in terms of the filter gain (or
% crossing 1 in terms of effective gain). When the intended impact is 0 the
% filter gain is 0... so no impact to signal because the filtered signal is
% attenuated to 0. Since filter gain changes exponentially so as to be
% linear in dB space, it is impossible to cross past 0 (from boosting to
% cutting for instance) via multiplication alone. To combat this challenge,
% this block enlists two rampers. When a single gain change involves
% crossing over the boost/cut boundary, the first ramper takes gain up yo
% the boundary and then the second ramper is set up to continue the journey
% on the other side of the boundary to ultimately reach the target impact
% gain.
%
% Inputs:
%   boost_max_db, cut_max_db: indicates maximum impact of tone impact in dB
%        which must be positive. A negative cut dB would imply a boost!
%   normalized_gain_impact : Target impact of the tone filter that must be
%        between -1 and 1. A value of "0" implies no effect, 1 and -1 are
%        maximum boost and cut respectively.
% Control Data:
%   FreezePhase(1) freezes the processing during this control operation
%   FreezePhase(2) indicates the current phase- always reset here to 1. The
%        phase indicates which of the two rampers is active. Once the first
%        ramper finishes, the second takes over (potentially to do
%        nothing if the adjustment did not require a boost/cut crossing)
%   Rampers(1) is the first phase ramper. Boost vs. cut is determined by
%        the sign of the linear current gain.
%   Rampers(2) is the second phase ramper. Boost vs. cut is determined by
%        the sign of the linear current gain.
%   *Note that the gain present in the rampers is the EFFECTIVE gain (aka
%   filter gain plus one).

% Step 4b: PHASES- Setup rampers for both phases
    % In order to have the desired ramp time, the slope must vary dependent
    % on the gain difference between target and current value.
    % Ramper's coefficient is therefore calculated as follows:
    %
    %   TargetGain = CurrentGain *( RampCoef ^ (Fs*RampTime_ms/1000) )
    %
    % therefore...
    %
    %                     log(TargetGain/CurrentGain)
    %   log(RampCoef) = ------------------------------
    %                        Fs*(RampTime_ms/1000)
    %

== matlab function BasicAudio_Target/BasicAudio/Volume/volume/InnerLink/Index2DbTable/lookup db from index ==
  data: volTableIdx input; volTabledB input; idx input; gain_value output; db_offset input int32; maxgain input
  events: trigger input FUNCTION_CALL_EVENT
function gain_value = LookupTheDB(volTableIdx, volTabledB, idx, db_offset, maxgain)
%#codegen
%
% Lookup volume table 
% Output Gain vlue from table
%

j = uint8(1);
gain_value = single(0.0);
interpolated_gain_dB=single(0.0);
interpolated_gain_dB_with_offset=single(0.0);

% workaround to type problem
idx = cast(idx, class(volTableIdx(end)));

%  bounds checking for vol - clip to max idx
if (idx > volTableIdx(end))
    idx = volTableIdx(end);
end
%  bounds checking for gain offset(No Boost) - clip to max offset level
if (db_offset > int32(maxgain))
    db_offset = int32(maxgain);
end
if (db_offset < int32(-10.0))
    db_offset = int32(-10.0);
end

% search through volume table to find index closest to vol
while (j <= numel(volTableIdx))
    if (idx <= volTableIdx(j))
        if (j <= 1)  % first indexed value is linearly interpolated to zero
            if (volTableIdx(j))
                percent = single(idx) / single(volTableIdx(j));
            else
                percent = single(1);
            end
            gain_value = percent * 10 ^ ( (volTabledB(j)+ single(db_offset)) / 20);
        else         % other values are interpolated in db space
            lastIdx = volTableIdx(j-1);
            percent = single(idx - lastIdx) / single(volTableIdx(j) - lastIdx);
            interpolated_gain_dB = (percent * (volTabledB(j) - volTabledB(j-1) ) ) + volTabledB(j-1);
            interpolated_gain_dB_with_offset= interpolated_gain_dB + single(db_offset); 
            gain_value = 10 ^ ( (interpolated_gain_dB_with_offset) / 20);            
        end
        break;
    else
        j = j + 1;
    end
end

== matlab function BasicAudio_Target/BasicAudio/Volume/volume/InnerLink/ramp parameters ==
  data rampRateRTC settings: description="If provided (i.e. non zero), this argument causes the \"ramp times (ms)\" input to be ignored. The block will calculate ramp times itself to ensure all gain changes happen at the db_per_sec slope provided."
  data rampTimeRTC settings: description=This vector signal must provide a linear target gain for every ramper.
  data rampTimeTune settings: description=|
      | The rampTimes_ms signal can accept one or more ramp times. If only one time is given, it is applied to all rampers. When more than one time is given, the times are delt out to the rampers in order. If not enough times are specified to cover all the rampers, the last given time is filled in to any remaining rampers.
      | NOTE: this input signal is entirely ignored if the db_per_sec input signal is non-zero. Attach the db_per_sec input to a ground block if you want to provide ramp times via this input.
  data rampTimeBounds settings: description="This input is required for control calculations to work. The \"Audio Stats\" block is a handy tool to lift this property right off an inbound audio signal and feed it to this block automatically without using workspace parameters or other constants."
  data rampRateBounds settings: description="This input is required for control calculations to work. The \"Audio Stats\" block is a handy tool to lift this property right off an inbound audio signal and feed it to this block automatically without using workspace parameters or other constants."
  data: rampRateRTC input; rampRate output; rampTimeRTC input; rampTimeTune input; ramptime output; rampTimeBounds parameter; rampRateBounds parameter
  events: trigger input FUNCTION_CALL_EVENT
function [rampRate, ramptime] = get_ramp_parameters(...
    rampRateRTC, rampTimeRTC, rampTimeTune,... % inputs
    rampTimeBounds, rampRateBounds) % parameters

% Ramp time and rate are provided to the block through RTC messages. However 
% in case neither of them are provided, the block will use the default ramp 
% time given in the tune variables.

    ramptime = single(rampTimeTune);
    rampRate = single(0);
    
    if (rampRateRTC)
        rampRate = single(rampRateRTC);
        rampRate = max(rampRateBounds(1), rampRate);
        rampRate = min(rampRateBounds(2), rampRate);
    end
    if (rampTimeRTC)
        ramptime = single(rampTimeRTC);
    end
    ramptime = max(rampTimeBounds(1), ramptime);
    ramptime = min(rampTimeBounds(2), ramptime);
end

== matlab function BasicAudio_Target/BasicAudio/Volume/volume/InnerLink/select one channel gain ==
  data: gainIn input; gainSingleChannel output
function gainSingleChannel = fcn(gainIn)
% Rgainy outputs gains of all channels. In the entertainment path, we only
% have one ramper meaning that the same gain gets applied to all channels.
% The following code extracts the gain of just the first channel as output.
    gainSingleChannel = squeeze(gainIn(:,1,:));
